simulink model "discrete_filter_1"  (Simulink 4.00)
settings: Solver=FixedStepDiscrete  StartTime=0.0  StopTime=10.0  RelTol=1e-3
settings Model: Creator=sofronis  LastModifiedBy=sofronis  AlgebraicLoopMsg=error  ExtModeAutoUpdateStatusClock=off  BooleanDataType=on

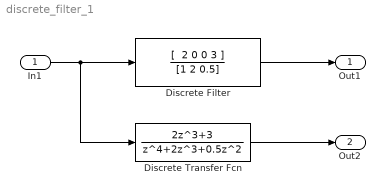
== system discrete_filter_1 ==
  In1 : Inport  Port=1  LatchInput=off  SampleTime=1
  Discrete Transfer Fcn : DiscreteTransferFcn  Numerator=[ 2 0 0 3]  Denominator=[1 2 0.5 0 0]  SampleTime=1  Realization=auto
      settings: RTWStateStorageClass=Auto
  Discrete Filter : DiscreteFilter  Numerator="[  2 0 0 3 ]"  Denominator=[1 2 0.5]  SampleTime=1  Realization=auto
      settings: RTWStateStorageClass=Auto
  Out1 : Outport  Port=1
  Out2 : Outport  Port=2
  wires:
  In1/1 -> Discrete Filter/1, Discrete Transfer Fcn/1
  Discrete Filter/1 -> Out1/1
  Discrete Transfer Fcn/1 -> Out2/1
